simulink model "myf_myr_extract"  (R2014a)
settings: Solver=ode1  StartTime=0.0  StopTime=15.7980  FixedStep=Tsample  RelTol=1e-3
settings Model: Creator=USER  LastModifiedBy=USER
settings DataIOCC: LimitDataPoints=off

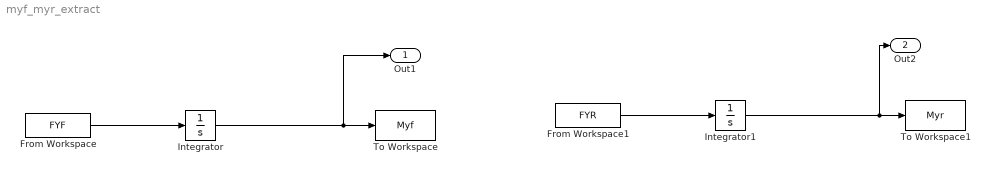
== system myf_myr_extract ==
  From Workspace : FromWorkspace  VariableName=FYF  SampleTime=0
  From Workspace1 : FromWorkspace  VariableName=FYR  SampleTime=0
  Integrator : Integrator
  Integrator1 : Integrator
  To Workspace : ToWorkspace  VariableName=Myf  SampleTime=-1
  To Workspace1 : ToWorkspace  VariableName=Myr  SampleTime=-1
  Out1 : Outport
  Out2 : Outport  Port=2
  wires:
  From Workspace/1 -> Integrator/1
  Integrator/1 -> Out1/1, To Workspace/1
  From Workspace1/1 -> Integrator1/1
  Integrator1/1 -> Out2/1, To Workspace1/1
